simulink model "IP_Sim"  (R2023b)
settings: Solver=FixedStepAuto  StartTime=0.0  StopTime=inf  FixedStep=0.01  RelTol=1e-3
InitFcn:
  | M = 0.5;
  | m = 0.5;
  | l = 0.3;
  | I = 0.006;
  | mu = 0.1;
  | g = 9.81
libraries: vrlib x2
settings Model: Creator=jitendra  LastModifiedBy=vcichella
settings DataIOCC: ExternalInput=getinputstruct(op_trim1)  InitialState=getstatestruct(op_trim1)  ReturnWorkspaceOutputs=off
settings OptimizationCC: ReuseModelBlockBuffer=off
settings DebuggingCC: UnconnectedInputMsg=warning  UnconnectedOutputMsg=warning  UnconnectedLineMsg=warning  ArithmeticOperatorsInVariantConditions=warning
settings ModelReferenceCC: EnableRefExpFcnMdlSchedulingChecks=on
settings SFSimCC: SimUseLocalCustomCode=off  CustomCodeUndefinedFunction=UseInterfaceOnly
settings RTWCC: RTWUseLocalCustomCode=off

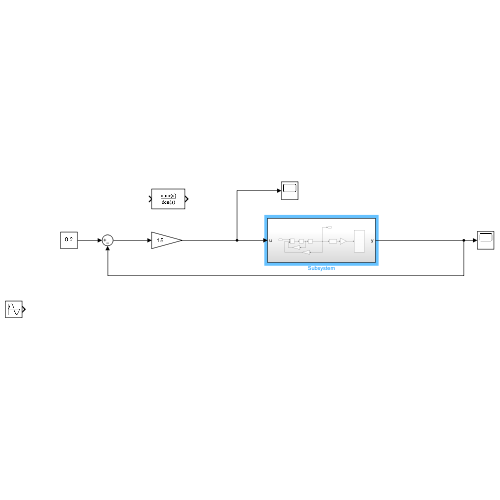
[thumbnail: Simulink's stored preview of the top-level diagram]
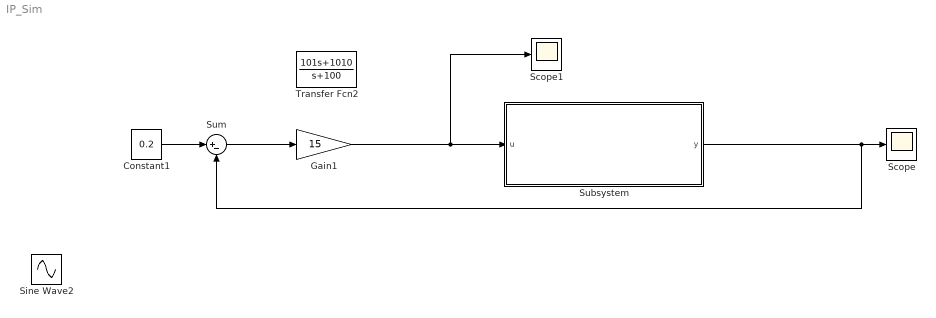
== system IP_Sim ==
  Constant1 : Constant  Value=0.2
  Gain1 : Gain  Gain=15
  Scope : Scope
  Scope1 : Scope
  Sine Wave2 : Sin  Amplitude=0.1  Frequency=0.5  SampleTime=0
  Subsystem : Subsystem
  Sum : Sum  Inputs=|+-
  Transfer Fcn2 : TransferFcn  Numerator=[101 1010]  Denominator=[1 100]
  wires:
  Sum/1 -> Gain1/1
  Constant1/1 -> Sum/1
  Gain1/1 -> Scope1/1, Subsystem/1(u)
  Subsystem/1(y) -> Sum/2, Scope/1

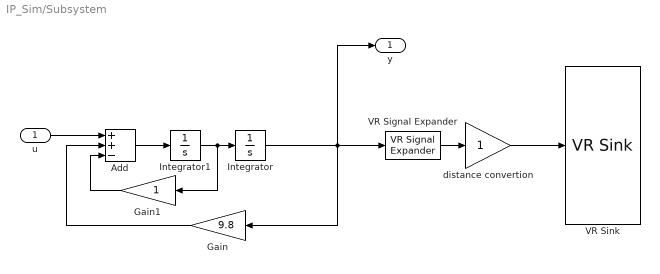
== system IP_Sim/Subsystem ==
  u : Inport
  Add : Sum  Inputs=++-
  Gain : Gain  Gain=9.8
  Gain1 : Gain
  Integrator : Integrator
  Integrator1 : Integrator
  VR Signal Expander : vrlib/VR Signal Expander  outwidth=4  outidx=[4]
  VR Sink : vrlib/VR Sink  InstantiateOnLoad=on  SampleTime=0.02  ViewEnable=on  RemoteChange=off  RemoteView=off  FieldsWritten=joint.rotation.4.1.1.double  WorldFileName=InvertedPendulum.wrl  AutoView=on  VideoDimensions=[]  AllowVariableSize=off
  distance convertion : Gain
  y : Outport
  wires:
  Add/1 -> Integrator1/1
  u/1 -> Add/1
  Integrator1/1 -> Gain1/1, Integrator/1
  Gain/1 -> Add/2
  VR Signal Expander/1 -> distance convertion/1
  Gain1/1 -> Add/3
  Integrator/1 -> Gain/1, y/1, VR Signal Expander/1
  distance convertion/1 -> VR Sink/1
